simulink model "chap7_13sim"  (Simulink 5.0)
settings: Solver=ode45  StartTime=0.0  StopTime=2  RelTol=1e-3
settings Model: LastModifiedBy=Administrator

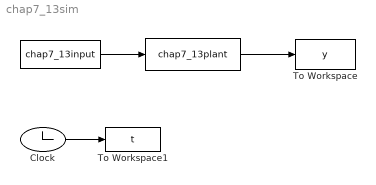
== system chap7_13sim ==
  " " : S-Function  FunctionName=chap7_13plant
  "  " : S-Function  FunctionName=chap7_13input
  Clock : Clock
      settings: Decimation=10
  To Workspace : ToWorkspace  VariableName=y  SampleTime=-1  SaveFormat=Array
  To Workspace1 : ToWorkspace  VariableName=t  SampleTime=-1  SaveFormat=Array
  wires:
  " "/1 -> To Workspace/1
  Clock/1 -> To Workspace1/1
  "  "/1 -> " "/1
